simulink model "casperdemo"  (Simulink 6.2)
settings: Solver=ode45  StartTime=0.0  StopTime=16384  RelTol=1e-3
libraries: xbsIndex_r3 x1645, casper_library x163, testbench_lib x15, xps_library x1
(part 12 of 12)

== system casperdemo/Complex FFT and PFB with multiple simultaneous inputs/fft/fft_biplex1/biplex_core/fft_stage_3/delay_b ==
  In1 : Inport  Port=1  LatchInput=off
  delay_slr : casper_library/Delays/delay_slr  DelayLen=2^(FFTSize-FFTStage)
  Out1 : Outport
  wires:
  In1/1 -> delay_slr/1
  delay_slr/1 -> Out1/1

== system casperdemo/Complex FFT and PFB with multiple simultaneous inputs/fft/fft_biplex1/biplex_core/fft_stage_3/delay_f ==
  In1 : Inport  Port=1  LatchInput=off
  delay_slr : casper_library/Delays/delay_slr  DelayLen=2^(FFTSize-FFTStage)
  Out1 : Outport
  wires:
  In1/1 -> delay_slr/1
  delay_slr/1 -> Out1/1

== system casperdemo/Real FFT and Real PFB/fft_biplex_real_4x/biplex_core/fft_stage_1/butterfly/c_to_ri ==
  c : Inport  Port=1  LatchInput=off
  Reinterpret : xbsIndex_r3/Reinterpret  force_arith_type=on  arith_type="Signed  (2's comp)"  force_bin_pt=on  bin_pt=BitWidth - 1  force_valid=on
  Reinterpret1 : xbsIndex_r3/Reinterpret  force_arith_type=on  arith_type="Signed  (2's comp)"  force_bin_pt=on  bin_pt=BitWidth - 1  force_valid=on
  Slice : xbsIndex_r3/Slice  mode=Upper Bit Location + Width  nbits=BitWidth  bit1=0  base1=MSB of Input  bit0=0  base0=LSB of Input  boolean_output=off  explicit_period=off  period=1  dbl_ovrd=off
  Slice1 : xbsIndex_r3/Slice  mode=Lower Bit Location + Width  nbits=BitWidth  bit1=0  base1=MSB of Input  bit0=0  base0=LSB of Input  boolean_output=off  explicit_period=off  period=1  dbl_ovrd=off
  re : Outport
  im : Outport  Port=2
  wires:
  Slice/1 -> Reinterpret/1
  Slice1/1 -> Reinterpret1/1
  Reinterpret/1 -> re/1
  Reinterpret1/1 -> im/1
  c/1 -> Slice/1, Slice1/1

== system casperdemo/Real FFT and Real PFB/fft_biplex_real_4x/biplex_core/fft_stage_1/butterfly/c_to_ri1 ==
  c : Inport  Port=1  LatchInput=off
  Reinterpret : xbsIndex_r3/Reinterpret  force_arith_type=on  arith_type="Signed  (2's comp)"  force_bin_pt=on  bin_pt=BitWidth - 1  force_valid=on
  Reinterpret1 : xbsIndex_r3/Reinterpret  force_arith_type=on  arith_type="Signed  (2's comp)"  force_bin_pt=on  bin_pt=BitWidth - 1  force_valid=on
  Slice : xbsIndex_r3/Slice  mode=Upper Bit Location + Width  nbits=BitWidth  bit1=0  base1=MSB of Input  bit0=0  base0=LSB of Input  boolean_output=off  explicit_period=off  period=1  dbl_ovrd=off
  Slice1 : xbsIndex_r3/Slice  mode=Lower Bit Location + Width  nbits=BitWidth  bit1=0  base1=MSB of Input  bit0=0  base0=LSB of Input  boolean_output=off  explicit_period=off  period=1  dbl_ovrd=off
  re : Outport
  im : Outport  Port=2
  wires:
  c/1 -> Slice1/1, Slice/1
  Reinterpret1/1 -> im/1
  Reinterpret/1 -> re/1
  Slice1/1 -> Reinterpret1/1
  Slice/1 -> Reinterpret/1

== system casperdemo/Real FFT and Real PFB/fft_biplex_real_4x/biplex_core/fft_stage_1/butterfly/ri_to_c ==
  re : Inport  Port=1  LatchInput=off
  im : Inport  Port=2  LatchInput=off
  Concat : xbsIndex_r3/Concat  num_inputs=2  explicit_period=off  period=1  dbl_ovrd=off
  Reinterpret : xbsIndex_r3/Reinterpret  force_arith_type=on  arith_type=Unsigned  force_bin_pt=on  bin_pt=0  force_valid=on
  Reinterpret1 : xbsIndex_r3/Reinterpret  force_arith_type=on  arith_type=Unsigned  force_bin_pt=on  bin_pt=0  force_valid=on
  c : Outport
  wires:
  Reinterpret/1 -> Concat/1
  Reinterpret1/1 -> Concat/2
  re/1 -> Reinterpret/1
  Concat/1 -> c/1
  im/1 -> Reinterpret1/1

== system casperdemo/Real FFT and Real PFB/fft_biplex_real_4x/biplex_core/fft_stage_1/butterfly/ri_to_c1 ==
  re : Inport  Port=1  LatchInput=off
  im : Inport  Port=2  LatchInput=off
  Concat : xbsIndex_r3/Concat  num_inputs=2  explicit_period=off  period=1  dbl_ovrd=off
  Reinterpret : xbsIndex_r3/Reinterpret  force_arith_type=on  arith_type=Unsigned  force_bin_pt=on  bin_pt=0  force_valid=on
  Reinterpret1 : xbsIndex_r3/Reinterpret  force_arith_type=on  arith_type=Unsigned  force_bin_pt=on  bin_pt=0  force_valid=on
  c : Outport
  wires:
  Reinterpret/1 -> Concat/1
  Reinterpret1/1 -> Concat/2
  re/1 -> Reinterpret/1
  Concat/1 -> c/1
  im/1 -> Reinterpret1/1

== system casperdemo/Real FFT and Real PFB/fft_biplex_real_4x/biplex_core/fft_stage_2/butterfly_direct/twiddle ==
  a : Inport  Port=1  LatchInput=off
  b : Inport  Port=2  LatchInput=off
  sync : Inport  Port=3  LatchInput=off
  twiddle_stage_2 : casper_library/FFTs/Twiddle/twiddle_stage_2  FFTSize=4  BitWidth=18  add_latency=2  mult_latency=3  bram_latency=2
  a_re : Outport
  a_im : Outport  Port=2
  bw_re : Outport  Port=3
  bw_im : Outport  Port=4
  sync_out : Outport  Port=5
  wires:
  a/1 -> twiddle_stage_2/1
  b/1 -> twiddle_stage_2/2
  sync/1 -> twiddle_stage_2/3
  twiddle_stage_2/1 -> a_re/1
  twiddle_stage_2/2 -> a_im/1
  twiddle_stage_2/3 -> bw_re/1
  twiddle_stage_2/4 -> bw_im/1
  twiddle_stage_2/5 -> sync_out/1

== system casperdemo/Real FFT and Real PFB/fft_biplex_real_4x/biplex_core/fft_stage_3/butterfly_direct/twiddle ==
  a : Inport  Port=1  LatchInput=off
  b : Inport  Port=2  LatchInput=off
  sync : Inport  Port=3  LatchInput=off
  twiddle_general_3mult : casper_library/FFTs/Twiddle/twiddle_general_3mult  Coeffs="[1+0i           6.1232e-017-1i               0.70711-0.70711i        -0.70711-0.70711i    ]"  StepPeriod=1  BitWidth=18  add_latency=2  mult_latency=3  bram_latency=2
  a_re : Outport
  a_im : Outport  Port=2
  bw_re : Outport  Port=3
  bw_im : Outport  Port=4
  sync_out : Outport  Port=5
  wires:
  a/1 -> twiddle_general_3mult/1
  b/1 -> twiddle_general_3mult/2
  sync/1 -> twiddle_general_3mult/3
  twiddle_general_3mult/1 -> a_re/1
  twiddle_general_3mult/2 -> a_im/1
  twiddle_general_3mult/3 -> bw_re/1
  twiddle_general_3mult/4 -> bw_im/1
  twiddle_general_3mult/5 -> sync_out/1

== system casperdemo/Real FFT and Real PFB/fft_biplex_real_4x/biplex_core/fft_stage_4/butterfly_direct/twiddle ==
  a : Inport  Port=1  LatchInput=off
  b : Inport  Port=2  LatchInput=off
  sync : Inport  Port=3  LatchInput=off
  twiddle_general_3mult : casper_library/FFTs/Twiddle/twiddle_general_3mult  Coeffs="[1+0i           6.1232e-017-1i               0.70711-0.70711i        -0.70711-0.70711i         0.92388-0.38268i        -0.38268-0.92388i         0.38268-0.92388i        -0.92388-0.38268i    ]"  StepPeriod=0  BitWidth=18  add_latency=2  mult_latency=3  bram_latency=2
  a_re : Outport
  a_im : Outport  Port=2
  bw_re : Outport  Port=3
  bw_im : Outport  Port=4
  sync_out : Outport  Port=5
  wires:
  a/1 -> twiddle_general_3mult/1
  b/1 -> twiddle_general_3mult/2
  sync/1 -> twiddle_general_3mult/3
  twiddle_general_3mult/1 -> a_re/1
  twiddle_general_3mult/2 -> a_im/1
  twiddle_general_3mult/3 -> bw_re/1
  twiddle_general_3mult/4 -> bw_im/1
  twiddle_general_3mult/5 -> sync_out/1

== system casperdemo/Complex FFT and PFB/fft/fft_biplex0/biplex_core/fft_stage_1/butterfly/c_to_ri ==
  c : Inport  Port=1  LatchInput=off
  Reinterpret : xbsIndex_r3/Reinterpret  force_arith_type=on  arith_type="Signed  (2's comp)"  force_bin_pt=on  bin_pt=BitWidth - 1  force_valid=on
  Reinterpret1 : xbsIndex_r3/Reinterpret  force_arith_type=on  arith_type="Signed  (2's comp)"  force_bin_pt=on  bin_pt=BitWidth - 1  force_valid=on
  Slice : xbsIndex_r3/Slice  mode=Upper Bit Location + Width  nbits=BitWidth  bit1=0  base1=MSB of Input  bit0=0  base0=LSB of Input  boolean_output=off  explicit_period=off  period=1  dbl_ovrd=off
  Slice1 : xbsIndex_r3/Slice  mode=Lower Bit Location + Width  nbits=BitWidth  bit1=0  base1=MSB of Input  bit0=0  base0=LSB of Input  boolean_output=off  explicit_period=off  period=1  dbl_ovrd=off
  re : Outport
  im : Outport  Port=2
  wires:
  Slice/1 -> Reinterpret/1
  Slice1/1 -> Reinterpret1/1
  Reinterpret/1 -> re/1
  Reinterpret1/1 -> im/1
  c/1 -> Slice/1, Slice1/1

== system casperdemo/Complex FFT and PFB/fft/fft_biplex0/biplex_core/fft_stage_1/butterfly/c_to_ri1 ==
  c : Inport  Port=1  LatchInput=off
  Reinterpret : xbsIndex_r3/Reinterpret  force_arith_type=on  arith_type="Signed  (2's comp)"  force_bin_pt=on  bin_pt=BitWidth - 1  force_valid=on
  Reinterpret1 : xbsIndex_r3/Reinterpret  force_arith_type=on  arith_type="Signed  (2's comp)"  force_bin_pt=on  bin_pt=BitWidth - 1  force_valid=on
  Slice : xbsIndex_r3/Slice  mode=Upper Bit Location + Width  nbits=BitWidth  bit1=0  base1=MSB of Input  bit0=0  base0=LSB of Input  boolean_output=off  explicit_period=off  period=1  dbl_ovrd=off
  Slice1 : xbsIndex_r3/Slice  mode=Lower Bit Location + Width  nbits=BitWidth  bit1=0  base1=MSB of Input  bit0=0  base0=LSB of Input  boolean_output=off  explicit_period=off  period=1  dbl_ovrd=off
  re : Outport
  im : Outport  Port=2
  wires:
  c/1 -> Slice1/1, Slice/1
  Reinterpret1/1 -> im/1
  Reinterpret/1 -> re/1
  Slice1/1 -> Reinterpret1/1
  Slice/1 -> Reinterpret/1

== system casperdemo/Complex FFT and PFB/fft/fft_biplex0/biplex_core/fft_stage_1/butterfly/ri_to_c ==
  re : Inport  Port=1  LatchInput=off
  im : Inport  Port=2  LatchInput=off
  Concat : xbsIndex_r3/Concat  num_inputs=2  explicit_period=off  period=1  dbl_ovrd=off
  Reinterpret : xbsIndex_r3/Reinterpret  force_arith_type=on  arith_type=Unsigned  force_bin_pt=on  bin_pt=0  force_valid=on
  Reinterpret1 : xbsIndex_r3/Reinterpret  force_arith_type=on  arith_type=Unsigned  force_bin_pt=on  bin_pt=0  force_valid=on
  c : Outport
  wires:
  Reinterpret/1 -> Concat/1
  Reinterpret1/1 -> Concat/2
  re/1 -> Reinterpret/1
  Concat/1 -> c/1
  im/1 -> Reinterpret1/1

== system casperdemo/Complex FFT and PFB/fft/fft_biplex0/biplex_core/fft_stage_1/butterfly/ri_to_c1 ==
  re : Inport  Port=1  LatchInput=off
  im : Inport  Port=2  LatchInput=off
  Concat : xbsIndex_r3/Concat  num_inputs=2  explicit_period=off  period=1  dbl_ovrd=off
  Reinterpret : xbsIndex_r3/Reinterpret  force_arith_type=on  arith_type=Unsigned  force_bin_pt=on  bin_pt=0  force_valid=on
  Reinterpret1 : xbsIndex_r3/Reinterpret  force_arith_type=on  arith_type=Unsigned  force_bin_pt=on  bin_pt=0  force_valid=on
  c : Outport
  wires:
  Reinterpret/1 -> Concat/1
  Reinterpret1/1 -> Concat/2
  re/1 -> Reinterpret/1
  Concat/1 -> c/1
  im/1 -> Reinterpret1/1

== system casperdemo/Complex FFT and PFB/fft/fft_biplex0/biplex_core/fft_stage_2/butterfly_direct/twiddle ==
  a : Inport  Port=1  LatchInput=off
  b : Inport  Port=2  LatchInput=off
  sync : Inport  Port=3  LatchInput=off
  twiddle_stage_2 : casper_library/FFTs/Twiddle/twiddle_stage_2  FFTSize=4  BitWidth=18  add_latency=2  mult_latency=3  bram_latency=2
  a_re : Outport
  a_im : Outport  Port=2
  bw_re : Outport  Port=3
  bw_im : Outport  Port=4
  sync_out : Outport  Port=5
  wires:
  a/1 -> twiddle_stage_2/1
  b/1 -> twiddle_stage_2/2
  sync/1 -> twiddle_stage_2/3
  twiddle_stage_2/1 -> a_re/1
  twiddle_stage_2/2 -> a_im/1
  twiddle_stage_2/3 -> bw_re/1
  twiddle_stage_2/4 -> bw_im/1
  twiddle_stage_2/5 -> sync_out/1

== system casperdemo/Complex FFT and PFB/fft/fft_biplex0/biplex_core/fft_stage_3/butterfly_direct/twiddle ==
  a : Inport  Port=1  LatchInput=off
  b : Inport  Port=2  LatchInput=off
  sync : Inport  Port=3  LatchInput=off
  twiddle_general_3mult : casper_library/FFTs/Twiddle/twiddle_general_3mult  Coeffs="[1+0i           6.1232e-017-1i               0.70711-0.70711i        -0.70711-0.70711i    ]"  StepPeriod=1  BitWidth=18  add_latency=2  mult_latency=3  bram_latency=2
  a_re : Outport
  a_im : Outport  Port=2
  bw_re : Outport  Port=3
  bw_im : Outport  Port=4
  sync_out : Outport  Port=5
  wires:
  a/1 -> twiddle_general_3mult/1
  b/1 -> twiddle_general_3mult/2
  sync/1 -> twiddle_general_3mult/3
  twiddle_general_3mult/1 -> a_re/1
  twiddle_general_3mult/2 -> a_im/1
  twiddle_general_3mult/3 -> bw_re/1
  twiddle_general_3mult/4 -> bw_im/1
  twiddle_general_3mult/5 -> sync_out/1

== system casperdemo/Complex FFT and PFB/fft/fft_biplex0/biplex_core/fft_stage_4/butterfly_direct/twiddle ==
  a : Inport  Port=1  LatchInput=off
  b : Inport  Port=2  LatchInput=off
  sync : Inport  Port=3  LatchInput=off
  twiddle_general_3mult : casper_library/FFTs/Twiddle/twiddle_general_3mult  Coeffs="[1+0i           6.1232e-017-1i               0.70711-0.70711i        -0.70711-0.70711i         0.92388-0.38268i        -0.38268-0.92388i         0.38268-0.92388i        -0.92388-0.38268i    ]"  StepPeriod=0  BitWidth=18  add_latency=2  mult_latency=3  bram_latency=2
  a_re : Outport
  a_im : Outport  Port=2
  bw_re : Outport  Port=3
  bw_im : Outport  Port=4
  sync_out : Outport  Port=5
  wires:
  a/1 -> twiddle_general_3mult/1
  b/1 -> twiddle_general_3mult/2
  sync/1 -> twiddle_general_3mult/3
  twiddle_general_3mult/1 -> a_re/1
  twiddle_general_3mult/2 -> a_im/1
  twiddle_general_3mult/3 -> bw_re/1
  twiddle_general_3mult/4 -> bw_im/1
  twiddle_general_3mult/5 -> sync_out/1

== system casperdemo/Complex FFT and PFB with multiple simultaneous inputs/fft/fft_biplex0/biplex_core/fft_stage_1/butterfly/c_to_ri ==
  c : Inport  Port=1  LatchInput=off
  Reinterpret : xbsIndex_r3/Reinterpret  force_arith_type=on  arith_type="Signed  (2's comp)"  force_bin_pt=on  bin_pt=BitWidth - 1  force_valid=on
  Reinterpret1 : xbsIndex_r3/Reinterpret  force_arith_type=on  arith_type="Signed  (2's comp)"  force_bin_pt=on  bin_pt=BitWidth - 1  force_valid=on
  Slice : xbsIndex_r3/Slice  mode=Upper Bit Location + Width  nbits=BitWidth  bit1=0  base1=MSB of Input  bit0=0  base0=LSB of Input  boolean_output=off  explicit_period=off  period=1  dbl_ovrd=off
  Slice1 : xbsIndex_r3/Slice  mode=Lower Bit Location + Width  nbits=BitWidth  bit1=0  base1=MSB of Input  bit0=0  base0=LSB of Input  boolean_output=off  explicit_period=off  period=1  dbl_ovrd=off
  re : Outport
  im : Outport  Port=2
  wires:
  c/1 -> Slice1/1, Slice/1
  Reinterpret1/1 -> im/1
  Reinterpret/1 -> re/1
  Slice1/1 -> Reinterpret1/1
  Slice/1 -> Reinterpret/1

== system casperdemo/Complex FFT and PFB with multiple simultaneous inputs/fft/fft_biplex0/biplex_core/fft_stage_1/butterfly/c_to_ri1 ==
  c : Inport  Port=1  LatchInput=off
  Reinterpret : xbsIndex_r3/Reinterpret  force_arith_type=on  arith_type="Signed  (2's comp)"  force_bin_pt=on  bin_pt=BitWidth - 1  force_valid=on
  Reinterpret1 : xbsIndex_r3/Reinterpret  force_arith_type=on  arith_type="Signed  (2's comp)"  force_bin_pt=on  bin_pt=BitWidth - 1  force_valid=on
  Slice : xbsIndex_r3/Slice  mode=Upper Bit Location + Width  nbits=BitWidth  bit1=0  base1=MSB of Input  bit0=0  base0=LSB of Input  boolean_output=off  explicit_period=off  period=1  dbl_ovrd=off
  Slice1 : xbsIndex_r3/Slice  mode=Lower Bit Location + Width  nbits=BitWidth  bit1=0  base1=MSB of Input  bit0=0  base0=LSB of Input  boolean_output=off  explicit_period=off  period=1  dbl_ovrd=off
  re : Outport
  im : Outport  Port=2
  wires:
  Slice/1 -> Reinterpret/1
  Slice1/1 -> Reinterpret1/1
  Reinterpret/1 -> re/1
  Reinterpret1/1 -> im/1
  c/1 -> Slice/1, Slice1/1

== system casperdemo/Complex FFT and PFB with multiple simultaneous inputs/fft/fft_biplex0/biplex_core/fft_stage_1/butterfly/ri_to_c ==
  re : Inport  Port=1  LatchInput=off
  im : Inport  Port=2  LatchInput=off
  Concat : xbsIndex_r3/Concat  num_inputs=2  explicit_period=off  period=1  dbl_ovrd=off
  Reinterpret : xbsIndex_r3/Reinterpret  force_arith_type=on  arith_type=Unsigned  force_bin_pt=on  bin_pt=0  force_valid=on
  Reinterpret1 : xbsIndex_r3/Reinterpret  force_arith_type=on  arith_type=Unsigned  force_bin_pt=on  bin_pt=0  force_valid=on
  c : Outport
  wires:
  im/1 -> Reinterpret1/1
  Concat/1 -> c/1
  re/1 -> Reinterpret/1
  Reinterpret1/1 -> Concat/2
  Reinterpret/1 -> Concat/1

== system casperdemo/Complex FFT and PFB with multiple simultaneous inputs/fft/fft_biplex0/biplex_core/fft_stage_1/butterfly/ri_to_c1 ==
  re : Inport  Port=1  LatchInput=off
  im : Inport  Port=2  LatchInput=off
  Concat : xbsIndex_r3/Concat  num_inputs=2  explicit_period=off  period=1  dbl_ovrd=off
  Reinterpret : xbsIndex_r3/Reinterpret  force_arith_type=on  arith_type=Unsigned  force_bin_pt=on  bin_pt=0  force_valid=on
  Reinterpret1 : xbsIndex_r3/Reinterpret  force_arith_type=on  arith_type=Unsigned  force_bin_pt=on  bin_pt=0  force_valid=on
  c : Outport
  wires:
  im/1 -> Reinterpret1/1
  Concat/1 -> c/1
  re/1 -> Reinterpret/1
  Reinterpret1/1 -> Concat/2
  Reinterpret/1 -> Concat/1

== system casperdemo/Complex FFT and PFB with multiple simultaneous inputs/fft/fft_biplex0/biplex_core/fft_stage_2/butterfly_direct/twiddle ==
  a : Inport  Port=1  LatchInput=off
  b : Inport  Port=2  LatchInput=off
  sync : Inport  Port=3  LatchInput=off
  twiddle_stage_2 : casper_library/FFTs/Twiddle/twiddle_stage_2  FFTSize=3  BitWidth=18  add_latency=2  mult_latency=3  bram_latency=2
  a_re : Outport
  a_im : Outport  Port=2
  bw_re : Outport  Port=3
  bw_im : Outport  Port=4
  sync_out : Outport  Port=5
  wires:
  a/1 -> twiddle_stage_2/1
  b/1 -> twiddle_stage_2/2
  sync/1 -> twiddle_stage_2/3
  twiddle_stage_2/1 -> a_re/1
  twiddle_stage_2/2 -> a_im/1
  twiddle_stage_2/3 -> bw_re/1
  twiddle_stage_2/4 -> bw_im/1
  twiddle_stage_2/5 -> sync_out/1

== system casperdemo/Complex FFT and PFB with multiple simultaneous inputs/fft/fft_biplex0/biplex_core/fft_stage_3/butterfly_direct/twiddle ==
  a : Inport  Port=1  LatchInput=off
  b : Inport  Port=2  LatchInput=off
  sync : Inport  Port=3  LatchInput=off
  twiddle_general_3mult : casper_library/FFTs/Twiddle/twiddle_general_3mult  Coeffs="[1+0i           6.1232e-017-1i               0.70711-0.70711i        -0.70711-0.70711i    ]"  StepPeriod=0  BitWidth=18  add_latency=2  mult_latency=3  bram_latency=2
  a_re : Outport
  a_im : Outport  Port=2
  bw_re : Outport  Port=3
  bw_im : Outport  Port=4
  sync_out : Outport  Port=5
  wires:
  a/1 -> twiddle_general_3mult/1
  b/1 -> twiddle_general_3mult/2
  sync/1 -> twiddle_general_3mult/3
  twiddle_general_3mult/1 -> a_re/1
  twiddle_general_3mult/2 -> a_im/1
  twiddle_general_3mult/3 -> bw_re/1
  twiddle_general_3mult/4 -> bw_im/1
  twiddle_general_3mult/5 -> sync_out/1

== system casperdemo/Complex FFT and PFB with multiple simultaneous inputs/fft/fft_biplex1/biplex_core/fft_stage_1/butterfly/c_to_ri ==
  c : Inport  Port=1  LatchInput=off
  Reinterpret : xbsIndex_r3/Reinterpret  force_arith_type=on  arith_type="Signed  (2's comp)"  force_bin_pt=on  bin_pt=BitWidth - 1  force_valid=on
  Reinterpret1 : xbsIndex_r3/Reinterpret  force_arith_type=on  arith_type="Signed  (2's comp)"  force_bin_pt=on  bin_pt=BitWidth - 1  force_valid=on
  Slice : xbsIndex_r3/Slice  mode=Upper Bit Location + Width  nbits=BitWidth  bit1=0  base1=MSB of Input  bit0=0  base0=LSB of Input  boolean_output=off  explicit_period=off  period=1  dbl_ovrd=off
  Slice1 : xbsIndex_r3/Slice  mode=Lower Bit Location + Width  nbits=BitWidth  bit1=0  base1=MSB of Input  bit0=0  base0=LSB of Input  boolean_output=off  explicit_period=off  period=1  dbl_ovrd=off
  re : Outport
  im : Outport  Port=2
  wires:
  Slice/1 -> Reinterpret/1
  Slice1/1 -> Reinterpret1/1
  Reinterpret/1 -> re/1
  Reinterpret1/1 -> im/1
  c/1 -> Slice/1, Slice1/1

== system casperdemo/Complex FFT and PFB with multiple simultaneous inputs/fft/fft_biplex1/biplex_core/fft_stage_1/butterfly/c_to_ri1 ==
  c : Inport  Port=1  LatchInput=off
  Reinterpret : xbsIndex_r3/Reinterpret  force_arith_type=on  arith_type="Signed  (2's comp)"  force_bin_pt=on  bin_pt=BitWidth - 1  force_valid=on
  Reinterpret1 : xbsIndex_r3/Reinterpret  force_arith_type=on  arith_type="Signed  (2's comp)"  force_bin_pt=on  bin_pt=BitWidth - 1  force_valid=on
  Slice : xbsIndex_r3/Slice  mode=Upper Bit Location + Width  nbits=BitWidth  bit1=0  base1=MSB of Input  bit0=0  base0=LSB of Input  boolean_output=off  explicit_period=off  period=1  dbl_ovrd=off
  Slice1 : xbsIndex_r3/Slice  mode=Lower Bit Location + Width  nbits=BitWidth  bit1=0  base1=MSB of Input  bit0=0  base0=LSB of Input  boolean_output=off  explicit_period=off  period=1  dbl_ovrd=off
  re : Outport
  im : Outport  Port=2
  wires:
  c/1 -> Slice1/1, Slice/1
  Reinterpret1/1 -> im/1
  Reinterpret/1 -> re/1
  Slice1/1 -> Reinterpret1/1
  Slice/1 -> Reinterpret/1

== system casperdemo/Complex FFT and PFB with multiple simultaneous inputs/fft/fft_biplex1/biplex_core/fft_stage_1/butterfly/ri_to_c ==
  re : Inport  Port=1  LatchInput=off
  im : Inport  Port=2  LatchInput=off
  Concat : xbsIndex_r3/Concat  num_inputs=2  explicit_period=off  period=1  dbl_ovrd=off
  Reinterpret : xbsIndex_r3/Reinterpret  force_arith_type=on  arith_type=Unsigned  force_bin_pt=on  bin_pt=0  force_valid=on
  Reinterpret1 : xbsIndex_r3/Reinterpret  force_arith_type=on  arith_type=Unsigned  force_bin_pt=on  bin_pt=0  force_valid=on
  c : Outport
  wires:
  Reinterpret/1 -> Concat/1
  Reinterpret1/1 -> Concat/2
  re/1 -> Reinterpret/1
  Concat/1 -> c/1
  im/1 -> Reinterpret1/1

== system casperdemo/Complex FFT and PFB with multiple simultaneous inputs/fft/fft_biplex1/biplex_core/fft_stage_1/butterfly/ri_to_c1 ==
  re : Inport  Port=1  LatchInput=off
  im : Inport  Port=2  LatchInput=off
  Concat : xbsIndex_r3/Concat  num_inputs=2  explicit_period=off  period=1  dbl_ovrd=off
  Reinterpret : xbsIndex_r3/Reinterpret  force_arith_type=on  arith_type=Unsigned  force_bin_pt=on  bin_pt=0  force_valid=on
  Reinterpret1 : xbsIndex_r3/Reinterpret  force_arith_type=on  arith_type=Unsigned  force_bin_pt=on  bin_pt=0  force_valid=on
  c : Outport
  wires:
  Reinterpret/1 -> Concat/1
  Reinterpret1/1 -> Concat/2
  re/1 -> Reinterpret/1
  Concat/1 -> c/1
  im/1 -> Reinterpret1/1

== system casperdemo/Complex FFT and PFB with multiple simultaneous inputs/fft/fft_biplex1/biplex_core/fft_stage_2/butterfly_direct/twiddle ==
  a : Inport  Port=1  LatchInput=off
  b : Inport  Port=2  LatchInput=off
  sync : Inport  Port=3  LatchInput=off
  twiddle_stage_2 : casper_library/FFTs/Twiddle/twiddle_stage_2  FFTSize=3  BitWidth=18  add_latency=2  mult_latency=3  bram_latency=2
  a_re : Outport
  a_im : Outport  Port=2
  bw_re : Outport  Port=3
  bw_im : Outport  Port=4
  sync_out : Outport  Port=5
  wires:
  a/1 -> twiddle_stage_2/1
  b/1 -> twiddle_stage_2/2
  sync/1 -> twiddle_stage_2/3
  twiddle_stage_2/1 -> a_re/1
  twiddle_stage_2/2 -> a_im/1
  twiddle_stage_2/3 -> bw_re/1
  twiddle_stage_2/4 -> bw_im/1
  twiddle_stage_2/5 -> sync_out/1

== system casperdemo/Complex FFT and PFB with multiple simultaneous inputs/fft/fft_biplex1/biplex_core/fft_stage_3/butterfly_direct/twiddle ==
  a : Inport  Port=1  LatchInput=off
  b : Inport  Port=2  LatchInput=off
  sync : Inport  Port=3  LatchInput=off
  twiddle_general_3mult : casper_library/FFTs/Twiddle/twiddle_general_3mult  Coeffs="[1+0i           6.1232e-017-1i               0.70711-0.70711i        -0.70711-0.70711i    ]"  StepPeriod=0  BitWidth=18  add_latency=2  mult_latency=3  bram_latency=2
  a_re : Outport
  a_im : Outport  Port=2
  bw_re : Outport  Port=3
  bw_im : Outport  Port=4
  sync_out : Outport  Port=5
  wires:
  a/1 -> twiddle_general_3mult/1
  b/1 -> twiddle_general_3mult/2
  sync/1 -> twiddle_general_3mult/3
  twiddle_general_3mult/1 -> a_re/1
  twiddle_general_3mult/2 -> a_im/1
  twiddle_general_3mult/3 -> bw_re/1
  twiddle_general_3mult/4 -> bw_im/1
  twiddle_general_3mult/5 -> sync_out/1
